simulink model "cartesianDifference"  (R2023a)
settings: Solver=ode4  StartTime=0.0  StopTime=10.0  FixedStep=6  RelTol=1e-3
settings Model: Creator=ndelurgio  LastModifiedBy=ndelurgio

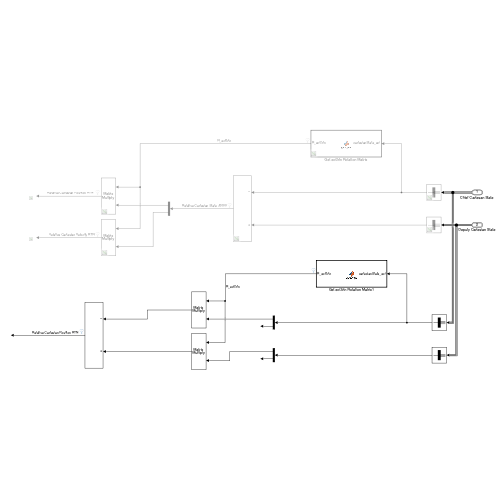
[thumbnail: Simulink's stored preview of the top-level diagram]
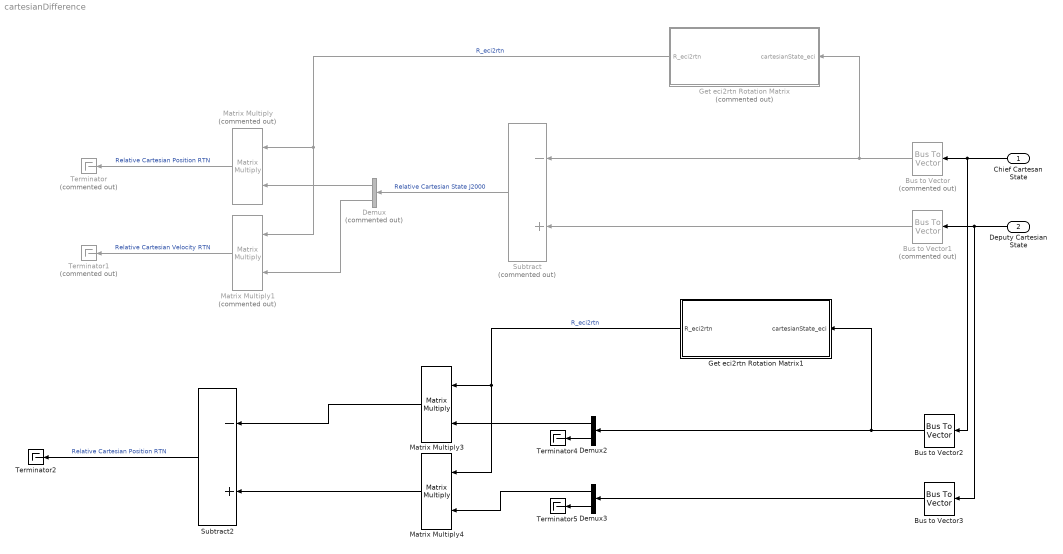
== system cartesianDifference ==
  Chief Cartesan State : Inport  OutDataTypeStr=Bus: cartesianState
  Deputy Cartesian State : Inport  Port=2  OutDataTypeStr=Bus: cartesianState
  Bus to Vector : BusToVector  Commented=on
  Bus to Vector1 : BusToVector  Commented=on
  Bus to Vector2 : BusToVector
  Bus to Vector3 : BusToVector
  Demux : Demux  Commented=on  Outputs=2
  Demux2 : Demux  Outputs=2
  Demux3 : Demux  Outputs=2
  Get eci2rtn Rotation Matrix : MATLAB Function  Commented=on  TreatAsAtomicUnit=on
  Get eci2rtn Rotation Matrix1 : MATLAB Function  TreatAsAtomicUnit=on
  Matrix Multiply : Product  Commented=on  Multiplication=Matrix(*)
  Matrix Multiply1 : Product  Commented=on  Multiplication=Matrix(*)
  Matrix Multiply3 : Product  Multiplication=Matrix(*)
  Matrix Multiply4 : Product  Multiplication=Matrix(*)
  Subtract : Sum  Commented=on  Inputs=-+
  Subtract2 : Sum  Inputs=-+
  Terminator : Terminator  Commented=on
  Terminator1 : Terminator  Commented=on
  Terminator2 : Terminator
  Terminator4 : Terminator
  Terminator5 : Terminator
  wires:
  Chief Cartesan State/1 -> Bus to Vector2/1, Bus to Vector/1
  Deputy Cartesian State/1 -> Bus to Vector3/1, Bus to Vector1/1
  Bus to Vector/1 -> Get eci2rtn Rotation Matrix/1(cartesianState_eci), Subtract/1
  Bus to Vector1/1 -> Subtract/2
  Subtract/1 -> Demux/1  "Relative Cartesian State J2000"
  Get eci2rtn Rotation Matrix/1(R_eci2rtn) -> Matrix Multiply1/1, Matrix Multiply/1  "R_eci2rtn"
  Matrix Multiply/1 -> Terminator/1  "Relative Cartesian Position RTN"
  Demux/1 -> Matrix Multiply/2
  Demux/2 -> Matrix Multiply1/2
  Matrix Multiply1/1 -> Terminator1/1  "Relative Cartesian Velocity RTN"
  Bus to Vector2/1 -> Demux2/1, Get eci2rtn Rotation Matrix1/1(cartesianState_eci)
  Bus to Vector3/1 -> Demux3/1
  Get eci2rtn Rotation Matrix1/1(R_eci2rtn) -> Matrix Multiply4/1, Matrix Multiply3/1  "R_eci2rtn"
  Demux2/2 -> Terminator4/1
  Demux2/1 -> Matrix Multiply3/2
  Demux3/2 -> Terminator5/1
  Demux3/1 -> Matrix Multiply4/2
  Matrix Multiply3/1 -> Subtract2/1
  Matrix Multiply4/1 -> Subtract2/2
  Subtract2/1 -> Terminator2/1  "Relative Cartesian Position RTN"

== matlab function cartesianDifference/Get eci2rtn Rotation Matrix ==
  data: cartesianState_eci input; R_eci2rtn output
function R_eci2rtn  = eci2rtn(cartesianState_eci)

[cartesianState_rtn, R_eci2rtn] = eci2rtn(cartesianState_eci);

end

== matlab function cartesianDifference/Get eci2rtn Rotation Matrix1 ==
  data: cartesianState_eci input; R_eci2rtn output
function R_eci2rtn  = eci2rtn(cartesianState_eci)

[cartesianState_rtn, R_eci2rtn] = eci2rtn(cartesianState_eci);

end
